simulink model "Exploration_pathplanner"  (R2015b)
settings: Solver=FixedStepAuto  StartTime=0.0  StopTime=inf  FixedStep=0.1  RelTol=1e-3
values from neighbouring files (symbols this model uses):
  Acoustic_Position = zeros(6,5)    [SetStuff256.m]
  GAPS = GAPS_found(i,:)    [ExplorationMain_original.m]
  n_acu = u(end,45)    [ExplorationMain.m]    (also in SetStuff256.m = 4)
undefined symbols (not defined in the file or in its folder): Data, Data_SL_Info
libraries: robotlib x13, realtime_pacer_lib x1
settings Model: Creator=einar  LastModifiedBy=saucer
settings OptimizationCC: OptimizeModelRefInitCode=on  LifeSpan=Inf  MaxStackSize=64
settings HardwareCC: ProdBitPerPointer=32  ProdLargestAtomicFloat=None  ProdIntDivRoundTo=Undefined  ProdEndianess=Unspecified  ProdWordSize=32  ProdHWDeviceType=Generic->Unspecified (assume 32-bit Generic)
settings RTWCC: SystemTargetFile=ert.tlc  TemplateMakefile=ert_default_tmf  Description=Embedded Coder  Toolchain=Catkin  TargetLang=C++
settings CodeAppCC: IgnoreCustomStorageClasses=off

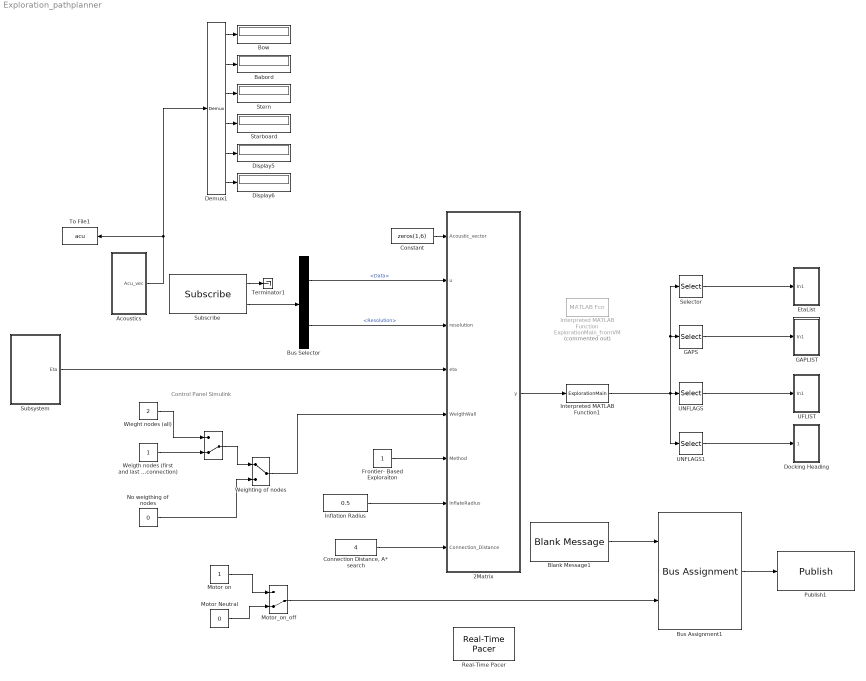
== system Exploration_pathplanner ==
  note: Control Panel Simulink
  " " : ManualSwitch  CurrentSetting=0
  "              Connection Distance, A* search" : Constant  Value=4  OutDataTypeStr=int8
  " Weighting of nodes" : ManualSwitch
  2Matrix : MATLAB Function  TreatAsAtomicUnit=on
  Acoustics : Subsystem
  Babord : Display
  Blank Message1 : robotlib/Blank Message  SourceLibraryInfo=This block requires Robotics System Toolbox  messageType=std_msgs/Bool  SampleTime=inf
  Bow : Display
  Bus Assignment1 : BusAssignment  AssignedSignals=Data
  Bus Selector : BusSelector  OutputSignals=Data,Info.Resolution
  Constant : Constant  Value=zeros(1,6)
  Demux1 : Demux  Outputs=6
  Display5 : Display
  Display6 : Display
  Docking Heading : Subsystem
  EtaList : Subsystem
  Frontier- Based Exploraiton : Constant
  GAPLIST : Subsystem
  GAPS : Selector  InputPortWidth=769  IndexOptions=Index vector (dialog)  Indices=[257:512]  OutputSizes=1
  Inflation Radius : Constant  Value=0.5
  Interpreted MATLAB Function : MATLABFcn  Commented=on  MATLABFcn=ExplorationMain_fromVM  OutputDimensions=769
  Interpreted MATLAB Function1 : MATLABFcn  MATLABFcn=ExplorationMain  OutputDimensions=769
  Motor Neutral : Constant  Value=0  OutDataTypeStr=boolean
  Motor on : Constant  OutDataTypeStr=boolean
  Motor_on_off : ManualSwitch  CurrentSetting=0
  No weigthing of nodes : Constant  Value=0
  Publish1 : robotlib/Publish  SourceLibraryInfo=This block requires Robotics System Toolbox  topicSource=Select from ROS network  topic=/Motor_on_off  messageType=std_msgs/Bool  messageQueueLength=1
  Real-Time Pacer : realtime_pacer_lib/Real-Time Pacer  simTimePerRealTime=1
  Selector : Selector  InputPortWidth=769  IndexOptions=Index vector (dialog)  Indices=[1:256]  OutputSizes=1
  Starboard : Display
  Stern : Display
  Subscribe : robotlib/Subscribe  SourceLibraryInfo=This block requires Robotics System Toolbox  topicSource=Select from ROS network  topic=/map  messageType=nav_msgs/OccupancyGrid  sampleTime=0.5  messageQueueLength=1
  Subsystem : Subsystem
  Terminator1 : Terminator
  To File1 : ToFile  Filename=acu  SaveFormat=Timeseries
  "UFLIST " : Subsystem
  UNFLAGS : Selector  InputPortWidth=769  IndexOptions=Index vector (dialog)  Indices=[513:768]  OutputSizes=1
  UNFLAGS1 : Selector  InputPortWidth=769  IndexOptions=Index vector (dialog)  Indices=[769]  OutputSizes=1
  Weigth nodes (first and last in connection) : Constant
  Wieght nodes (all) : Constant  Value=2
  wires:
  Subscribe/2 -> Bus Selector/1
  Bus Selector/1 -> 2Matrix/2(u)  "<Data>"
  2Matrix/1(y) -> Interpreted MATLAB Function1/1
  Bus Selector/2 -> 2Matrix/3(resolution)  "<Resolution>"
  " Weighting of nodes"/1 -> 2Matrix/5(WeigthWall)
  Weigth nodes (first and last in connection)/1 -> " "/2
  No weigthing of nodes/1 -> " Weighting of nodes"/2
  Frontier- Based Exploraiton/1 -> 2Matrix/6(Method)
  Selector/1 -> EtaList/1(In1)
  GAPS/1 -> GAPLIST/1(In1)
  UNFLAGS/1 -> "UFLIST "/1(In1)
  " "/1 -> " Weighting of nodes"/1
  Wieght nodes (all)/1 -> " "/1
  Inflation Radius/1 -> 2Matrix/7(InflateRadius)
  "              Connection Distance, A* search"/1 -> 2Matrix/8(Connection_Distance)
  Bus Assignment1/1 -> Publish1/1
  Blank Message1/1 -> Bus Assignment1/1
  Motor_on_off/1 -> Bus Assignment1/2
  Motor Neutral/1 -> Motor_on_off/2
  Motor on/1 -> Motor_on_off/1
  Subscribe/1 -> Terminator1/1
  Subsystem/1(Eta) -> 2Matrix/4(eta)
  Acoustics/1(Acu_vec) -> Demux1/1, To File1/1
  Demux1/1 -> Bow/1
  Demux1/2 -> Babord/1
  Demux1/3 -> Stern/1
  Demux1/4 -> Starboard/1
  Demux1/5 -> Display5/1
  Demux1/6 -> Display6/1
  Interpreted MATLAB Function1/1 -> Selector/1, GAPS/1, UNFLAGS1/1, UNFLAGS/1
  UNFLAGS1/1 -> Docking Heading/1(Docking Psi)
  Constant/1 -> 2Matrix/1(Acoustic_vector)

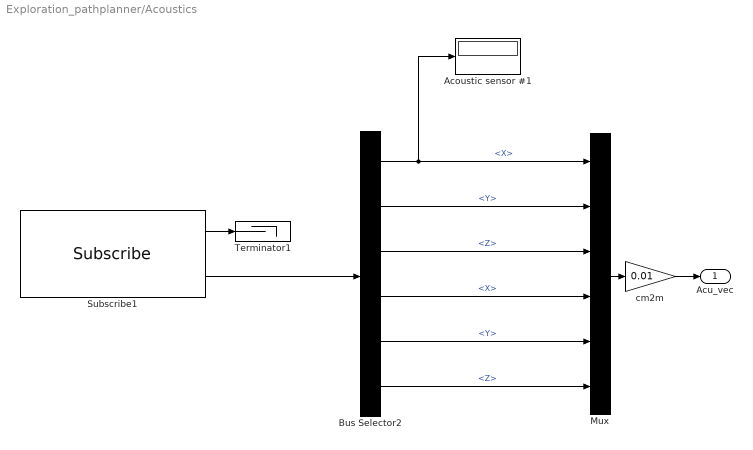
== system Exploration_pathplanner/Acoustics ==
  Acoustic sensor #1 : Display
  Bus Selector2 : BusSelector  OutputSignals=Linear.X,Linear.Y,Linear.Z,Angular.X,Angular.Y,Angular.Z
  Mux : Mux  Inputs=6
  Subscribe1 : robotlib/Subscribe  SourceLibraryInfo=This block requires Robotics System Toolbox  topicSource=Select from ROS network  topic=/Acoustics  messageType=geometry_msgs/Twist  sampleTime=-1  messageQueueLength=1
  Terminator1 : Terminator
  cm2m : Gain  Gain=0.01
  Acu_vec : Outport
  wires:
  Subscribe1/1 -> Terminator1/1
  Subscribe1/2 -> Bus Selector2/1
  Bus Selector2/1 -> Mux/1, Acoustic sensor #1/1  "<X>"
  Bus Selector2/6 -> Mux/6  "<Z>"
  Bus Selector2/5 -> Mux/5  "<Y>"
  Bus Selector2/4 -> Mux/4  "<X>"
  Bus Selector2/3 -> Mux/3  "<Z>"
  Bus Selector2/2 -> Mux/2  "<Y>"
  Mux/1 -> cm2m/1
  cm2m/1 -> Acu_vec/1

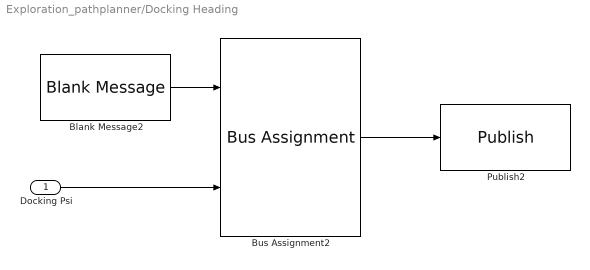
== system Exploration_pathplanner/Docking Heading ==
  Docking Psi : Inport
  Blank Message2 : robotlib/Blank Message  SourceLibraryInfo=This block requires Robotics System Toolbox  messageType=std_msgs/Float64  SampleTime=inf
  Bus Assignment2 : BusAssignment  AssignedSignals=Data
  Publish2 : robotlib/Publish  SourceLibraryInfo=This block requires Robotics System Toolbox  topicSource=Specify your own  topic=/Docking_heading  messageType=std_msgs/Float64  messageQueueLength=1
  wires:
  Blank Message2/1 -> Bus Assignment2/1
  Bus Assignment2/1 -> Publish2/1
  Docking Psi/1 -> Bus Assignment2/2

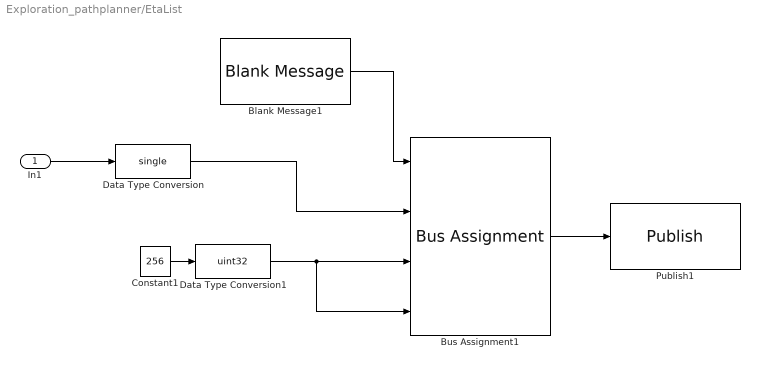
== system Exploration_pathplanner/EtaList ==
  In1 : Inport
  Blank Message1 : robotlib/Blank Message  SourceLibraryInfo=This block requires Robotics System Toolbox  messageType=std_msgs/Float32MultiArray  SampleTime=inf
  Bus Assignment1 : BusAssignment  AssignedSignals=Data,Data_SL_Info.CurrentLength,Data_SL_Info.ReceivedLength
  Constant1 : Constant  Value=256
  Data Type Conversion : DataTypeConversion  OutDataTypeStr=single
  Data Type Conversion1 : DataTypeConversion  OutDataTypeStr=uint32
  Publish1 : robotlib/Publish  SourceLibraryInfo=This block requires Robotics System Toolbox  topicSource=Specify your own  topic=/Path  messageType=std_msgs/Float32MultiArray  messageQueueLength=1
  wires:
  Constant1/1 -> Data Type Conversion1/1
  Data Type Conversion/1 -> Bus Assignment1/2
  Bus Assignment1/1 -> Publish1/1
  Blank Message1/1 -> Bus Assignment1/1
  Data Type Conversion1/1 -> Bus Assignment1/4, Bus Assignment1/3
  In1/1 -> Data Type Conversion/1

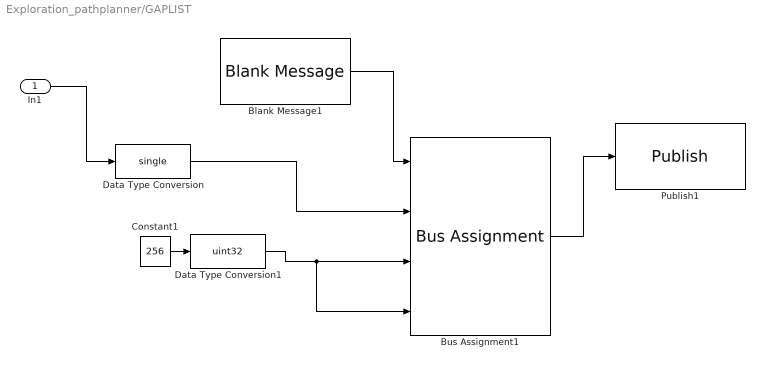
== system Exploration_pathplanner/GAPLIST ==
  In1 : Inport
  Blank Message1 : robotlib/Blank Message  SourceLibraryInfo=This block requires Robotics System Toolbox  messageType=std_msgs/Float32MultiArray  SampleTime=inf
  Bus Assignment1 : BusAssignment  AssignedSignals=Data,Data_SL_Info.CurrentLength,Data_SL_Info.ReceivedLength
  Constant1 : Constant  Value=256
  Data Type Conversion : DataTypeConversion  OutDataTypeStr=single
  Data Type Conversion1 : DataTypeConversion  OutDataTypeStr=uint32
  Publish1 : robotlib/Publish  SourceLibraryInfo=This block requires Robotics System Toolbox  topicSource=Specify your own  topic=/GAPS  messageType=std_msgs/Float32MultiArray  messageQueueLength=1
  wires:
  In1/1 -> Data Type Conversion/1
  Data Type Conversion1/1 -> Bus Assignment1/3, Bus Assignment1/4
  Blank Message1/1 -> Bus Assignment1/1
  Bus Assignment1/1 -> Publish1/1
  Data Type Conversion/1 -> Bus Assignment1/2
  Constant1/1 -> Data Type Conversion1/1

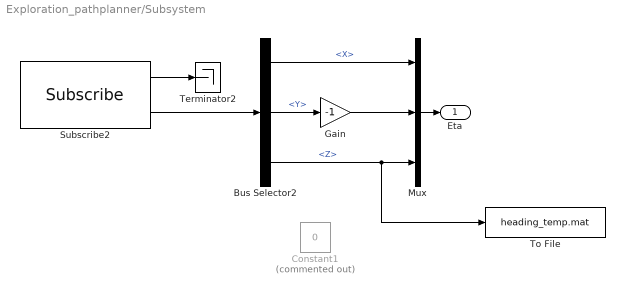
== system Exploration_pathplanner/Subsystem ==
  Bus Selector2 : BusSelector  OutputSignals=X,Y,Z
  Constant1 : Constant  Commented=on  Value=0
  Gain : Gain  Gain=-1
  Mux : Mux  Inputs=3
  Subscribe2 : robotlib/Subscribe  SourceLibraryInfo=This block requires Robotics System Toolbox  topicSource=Specify your own  topic=/Position  messageType=geometry_msgs/Vector3  sampleTime=-1  messageQueueLength=1
  Terminator2 : Terminator
  To File : ToFile  Filename=heading_temp.mat  SaveFormat=Timeseries
  Eta : Outport
  wires:
  Bus Selector2/1 -> Mux/1  "<X>"
  Subscribe2/2 -> Bus Selector2/1
  Mux/1 -> Eta/1
  Subscribe2/1 -> Terminator2/1
  Bus Selector2/2 -> Gain/1  "<Y>"
  Bus Selector2/3 -> To File/1, Mux/3  "<Z>"
  Gain/1 -> Mux/2

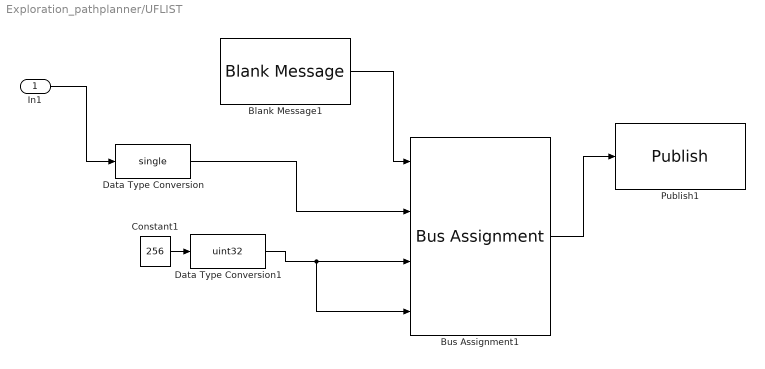
== system Exploration_pathplanner/UFLIST  ==
  In1 : Inport
  Blank Message1 : robotlib/Blank Message  SourceLibraryInfo=This block requires Robotics System Toolbox  messageType=std_msgs/Float32MultiArray  SampleTime=inf
  Bus Assignment1 : BusAssignment  AssignedSignals=Data,Data_SL_Info.CurrentLength,Data_SL_Info.ReceivedLength
  Constant1 : Constant  Value=256
  Data Type Conversion : DataTypeConversion  OutDataTypeStr=single
  Data Type Conversion1 : DataTypeConversion  OutDataTypeStr=uint32
  Publish1 : robotlib/Publish  SourceLibraryInfo=This block requires Robotics System Toolbox  topicSource=Specify your own  topic=/UNFGAPS  messageType=std_msgs/Float32MultiArray  messageQueueLength=1
  wires:
  Constant1/1 -> Data Type Conversion1/1
  Data Type Conversion/1 -> Bus Assignment1/2
  Bus Assignment1/1 -> Publish1/1
  Blank Message1/1 -> Bus Assignment1/1
  Data Type Conversion1/1 -> Bus Assignment1/4, Bus Assignment1/3
  In1/1 -> Data Type Conversion/1

== matlab function Exploration_pathplanner/2Matrix ==
  data: n_acu parameter; Acoustic_Position parameter; Acoustic_vector input; u input; resolution input; y output; eta input; WeigthWall input; Method input; InflateRadius input; Connection_Distance input
function y  = fcn(n_acu,Acoustic_Position,Acoustic_vector,u,resolution,eta,WeigthWall,Method,InflateRadius,Connection_Distance)
%% Added
%eta(3)=0;
%%
K=length(u)^0.5;
y=zeros(K+1,K);
MAP=zeros(K+1,K);
for i=1:K;
    MAP(i,1:K)=u((i-1)*K+1:i*K);
end
MAP(K+1,1:3)=eta;
MAP(K+1,4)=resolution;
MAP(K+1,5)=WeigthWall;
MAP(K+1,6)=Method;
MAP(K+1,7)=InflateRadius;
MAP(K+1,8)=Connection_Distance;
%% Acoustics
for i = 1:length(Acoustic_vector)
    MAP(K+1,8+i) = Acoustic_vector(i);
end
MAP(K+1,15:44) = reshape(Acoustic_Position',[1,6*5]);
MAP(K+1,45) = n_acu;
%%

y = (MAP);
